simulink model "plantaClosedLoop"  (R2022b)
settings: Solver=VariableStepAuto  StartTime=0.0  StopTime=10.0  MaxStep=0.01  RelTol=1e-3
values from neighbouring files (symbols this model uses):
  d1 = 130.75e-3    (= 0.13075)    [FoundTF.m]    (also in TF.mat)
  d2 = 50.75e-3    (= 0.05075)    [FoundTF.m]    (also in TF.mat)
  DZ = 3    [FoundTF.m]    (also in TF.mat)
  Gden = cell2mat(G.Denominator)    [FoundTF.m]    (also in TF.mat = [1 3.334 0])
  Gnum = cell2mat(G.Numerator)    [FoundTF.m]    (also in TF.mat = [0 0 1.02856666667])
  I = 15e-5    (= 0.00015)    [FoundTF.m]    (also in TF.mat)
  MAX_PWM = 80    [FoundTF.m]    (also in TF.mat)
  thetap = 90    [TF.mat]
  wb = 0.105948    [FoundTF.m]    (also in TF.mat)
  wcp = 0.014145    [FoundTF.m]    (also in TF.mat)
  wm = 0.030411    [FoundTF.m]    (also in TF.mat)
undefined symbols (not defined in the file or in its folder): b, PWM_INPUT
libraries: slpidlib x6
settings Model: Creator=felip  LastModifiedBy=felip

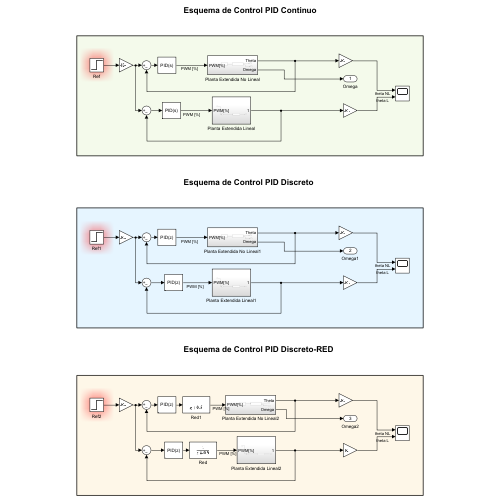
[thumbnail: Simulink's stored preview of the top-level diagram]
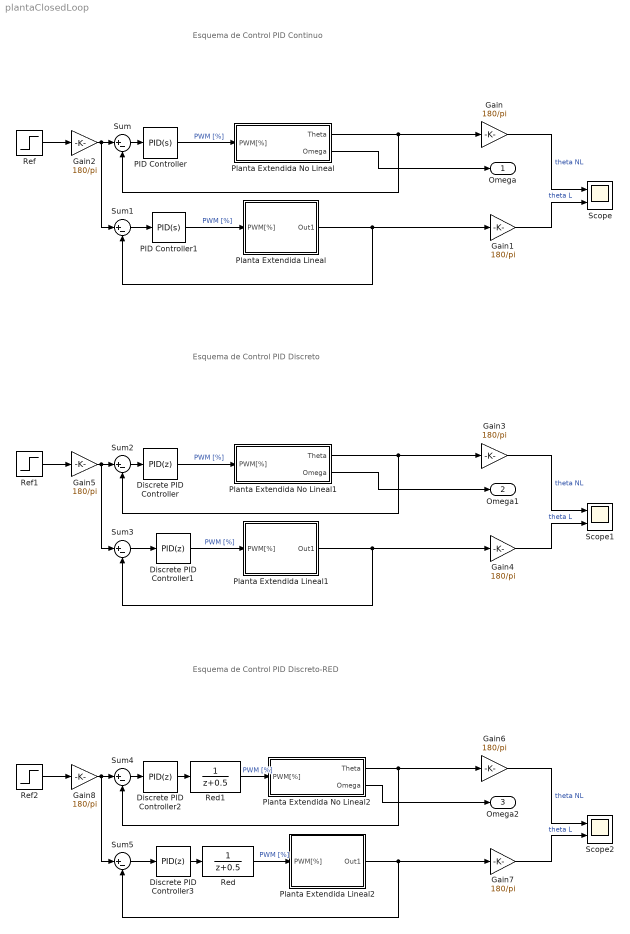
== system plantaClosedLoop ==
  note: Esquema de Control PID Continuo
  note: Esquema de Control PID Discreto
  note: Esquema de Control PID Discreto-RED
  Discrete PID Controller{,1..3} (4 alike) : slpidlib/PID Controller  Controller=PID  Form=Parallel  TimeDomain=Discrete-time  UseExternalTs=off  SampleTime=-1  IntegratorMethod=Forward Euler  FilterMethod=Forward Euler  ControllerParametersSource=internal  P=1  I=1  UseKiTs=off  D=0  N=100  UseFilter=on  TunerSelectOption=Transfer Function Based (PID Tuner App)  InitialConditionSource=internal  InitialConditionForIntegrator=0  InitialConditionForFilter=0  DifferentiatorICPrevScaledInput=0  ExternalReset=none  TrackingMode=off  Kt=1  LimitOutput=off  SatLimitsSource=internal  UpperSaturationLimit=inf  LowerSaturationLimit=-inf  LinearizeAsGain=off  AntiWindupMode=none  Kb=1  LimitIntegrator=off  UpperIntegratorSaturationLimit=inf  LowerIntegratorSaturationLimit=-inf  POutMin=[]  POutMax=[]  IOutMin=[]  IOutMax=[]  DOutMin=[]  DOutMax=[]  NOutMin=[]  NOutMax=[]  SumOutMin=[]  SumOutMax=[]  SaturationOutMin=[]  SaturationOutMax=[]  PParamMin=[]  PParamMax=[]  IParamMin=[]  IParamMax=[]  DParamMin=[]  DParamMax=[]  NParamMin=[]  NParamMax=[]  KbParamMin=[]  KbParamMax=[]  KtParamMin=[]  KtParamMax=[]  KbOutMin=[]  KbOutMax=[]  KtOutMin=[]  KtOutMax=[]  IntegratorOutMin=[]  IntegratorOutMax=[]  FilterOutMin=[]  FilterOutMax=[]  SumI1OutMin=[]  SumI1OutMax=[]  SumI2OutMin=[]  SumI2OutMax=[]  SumI3OutMin=[]  SumI3OutMax=[]  SumI4OutMin=[]  SumI4OutMax=[]  SumDOutMin=[]  SumDOutMax=[]  DifferentiatorOutMin=[]  DifferentiatorOutMax=[]  FilterDiffOutCoefMin=[]  FilterDiffOutCoefMax=[]  ReciprocalOutMin=[]  ReciprocalOutMax=[]  SumDenOutMin=[]  SumDenOutMax=[]  SumNumOutMin=[]  SumNumOutMax=[]  DivideOutMin=[]  DivideOutMax=[]  UdiffTsProdOutMin=[]  UdiffTsProdOutMax=[]  NTsProdOutMin=[]  NTsProdOutMax=[]  UintegralTsProdOutMin=[]  UintegralTsProdOutMax=[]  UngainTsProdOutMin=[]  UngainTsProdOutMax=[]  ClampingZeroOutDataTypeStr=Inherit: Inherit via back propagation  ClampingZeroOutMin=[]  ClampingZeroOutMax=[]  FilterDenConstantOutDataTypeStr=Inherit: Inherit via back propagation  FilterDenConstantOutMin=[]  FilterDenConstantOutMax=[]  PCopyOutDataTypeStr=Inherit: Inherit via back propagation  PCopyOutMin=[]  PCopyOutMax=[]  NCopyOutDataTypeStr=Inherit: Inherit via back propagation  NCopyOutMin=[]  NCopyOutMax=[]  IntegratorContinuousStateAttributes=''  IntegratorStateMustResolveToSignalObject=off  IntegratorRTWStateStorageClass=Auto  FilterContinuousStateAttributes=''  FilterStateMustResolveToSignalObject=off  FilterRTWStateStorageClass=Auto  ParallelPVariant=InternalParameters  IdealPVariant=Disabled  IVariant=InternalParameters  DVariant=InternalParameters  IntegratorVariant=Discrete  SatVariant=Disabled  AWVariant=Passthrough  PCopyVariant=Disabled  TRVariant=Disabled  FdbkBlocksVariant=Forward  IdealPFdbkVariant=Disabled  SatFdbkVariant=Disabled  DerivativeFilterVariant=ForwardEulerFilter  NVariant=InternalParameters  NCopyVariant=Disabled  FilterICVariant=InternalICsFilter  IntegratorICVariant=InternalICs  ExternalResetVariant=Disabled  TRSumVariant=Passthrough  SumFdbkVariant=Disabled  SumVariant=Sum_PID  TsampFilterVariant=InternalTs  TsampNgainVariant=Passthrough  TsampIntegralVariant=Passthrough  ExternalSaturationOutDataTypeStr=Inherit: Same as second input
      settings: LibrarySourceBlock=simulink/Discrete/Discrete PID Controller
  Gain{,1..8} (9 alike) : Gain  Gain=180/pi
  PID Controller : slpidlib/PID Controller  Controller=PID  Form=Parallel  TimeDomain=Continuous-time  UseExternalTs=off  SampleTime=-1  IntegratorMethod=Forward Euler  FilterMethod=Forward Euler  ControllerParametersSource=internal  P=1  I=1  UseKiTs=off  D=0  N=100  UseFilter=on  TunerSelectOption=Transfer Function Based (PID Tuner App)  InitialConditionSource=internal  InitialConditionForIntegrator=0  InitialConditionForFilter=0  DifferentiatorICPrevScaledInput=0  ExternalReset=none  TrackingMode=off  Kt=1  LimitOutput=off  SatLimitsSource=internal  UpperSaturationLimit=inf  LowerSaturationLimit=-inf  LinearizeAsGain=on  AntiWindupMode=none  Kb=1  LimitIntegrator=off  UpperIntegratorSaturationLimit=inf  LowerIntegratorSaturationLimit=-inf  POutMin=[]  POutMax=[]  IOutMin=[]  IOutMax=[]  DOutMin=[]  DOutMax=[]  NOutMin=[]  NOutMax=[]  SumOutMin=[]  SumOutMax=[]  SaturationOutMin=[]  SaturationOutMax=[]  PParamMin=[]  PParamMax=[]  IParamMin=[]  IParamMax=[]  DParamMin=[]  DParamMax=[]  NParamMin=[]  NParamMax=[]  KbParamMin=[]  KbParamMax=[]  KtParamMin=[]  KtParamMax=[]  KbOutMin=[]  KbOutMax=[]  KtOutMin=[]  KtOutMax=[]  IntegratorOutMin=[]  IntegratorOutMax=[]  FilterOutMin=[]  FilterOutMax=[]  SumI1OutMin=[]  SumI1OutMax=[]  SumI2OutMin=[]  SumI2OutMax=[]  SumI3OutMin=[]  SumI3OutMax=[]  SumI4OutMin=[]  SumI4OutMax=[]  SumDOutMin=[]  SumDOutMax=[]  DifferentiatorOutMin=[]  DifferentiatorOutMax=[]  FilterDiffOutCoefMin=[]  FilterDiffOutCoefMax=[]  ReciprocalOutMin=[]  ReciprocalOutMax=[]  SumDenOutMin=[]  SumDenOutMax=[]  SumNumOutMin=[]  SumNumOutMax=[]  DivideOutMin=[]  DivideOutMax=[]  UdiffTsProdOutMin=[]  UdiffTsProdOutMax=[]  NTsProdOutMin=[]  NTsProdOutMax=[]  UintegralTsProdOutMin=[]  UintegralTsProdOutMax=[]  UngainTsProdOutMin=[]  UngainTsProdOutMax=[]  ClampingZeroOutDataTypeStr=Inherit: Inherit via back propagation  ClampingZeroOutMin=[]  ClampingZeroOutMax=[]  FilterDenConstantOutDataTypeStr=Inherit: Inherit via back propagation  FilterDenConstantOutMin=[]  FilterDenConstantOutMax=[]  PCopyOutDataTypeStr=Inherit: Inherit via back propagation  PCopyOutMin=[]  PCopyOutMax=[]  NCopyOutDataTypeStr=Inherit: Inherit via back propagation  NCopyOutMin=[]  NCopyOutMax=[]  IntegratorContinuousStateAttributes=''  IntegratorStateMustResolveToSignalObject=off  IntegratorRTWStateStorageClass=Auto  FilterContinuousStateAttributes=''  FilterStateMustResolveToSignalObject=off  FilterRTWStateStorageClass=Auto  ParallelPVariant=InternalParameters  IdealPVariant=Disabled  IVariant=InternalParameters  DVariant=InternalParameters  IntegratorVariant=Continuous  SatVariant=Disabled  AWVariant=Passthrough  PCopyVariant=Disabled  TRVariant=Disabled  FdbkBlocksVariant=Forward  IdealPFdbkVariant=Disabled  SatFdbkVariant=Disabled  DerivativeFilterVariant=ContFilter  NVariant=InternalParameters  NCopyVariant=Disabled  FilterICVariant=InternalICsFilter  IntegratorICVariant=InternalICs  ExternalResetVariant=Disabled  TRSumVariant=Passthrough  SumFdbkVariant=Disabled  SumVariant=Sum_PID  TsampFilterVariant=InternalTs  TsampNgainVariant=Passthrough  TsampIntegralVariant=Passthrough  ExternalSaturationOutDataTypeStr=Inherit: Same as second input
  PID Controller1 : slpidlib/PID Controller  Controller=PID  Form=Parallel  TimeDomain=Continuous-time  UseExternalTs=off  SampleTime=-1  IntegratorMethod=Forward Euler  FilterMethod=Forward Euler  ControllerParametersSource=internal  P=1  I=1  UseKiTs=off  D=0  N=100  UseFilter=on  TunerSelectOption=Transfer Function Based (PID Tuner App)  InitialConditionSource=internal  InitialConditionForIntegrator=0  InitialConditionForFilter=0  DifferentiatorICPrevScaledInput=0  ExternalReset=none  TrackingMode=off  Kt=1  LimitOutput=off  SatLimitsSource=internal  UpperSaturationLimit=inf  LowerSaturationLimit=-inf  LinearizeAsGain=on  AntiWindupMode=none  Kb=1  LimitIntegrator=off  UpperIntegratorSaturationLimit=inf  LowerIntegratorSaturationLimit=-inf  POutMin=[]  POutMax=[]  IOutMin=[]  IOutMax=[]  DOutMin=[]  DOutMax=[]  NOutMin=[]  NOutMax=[]  SumOutMin=[]  SumOutMax=[]  SaturationOutMin=[]  SaturationOutMax=[]  PParamMin=[]  PParamMax=[]  IParamMin=[]  IParamMax=[]  DParamMin=[]  DParamMax=[]  NParamMin=[]  NParamMax=[]  KbParamMin=[]  KbParamMax=[]  KtParamMin=[]  KtParamMax=[]  KbOutMin=[]  KbOutMax=[]  KtOutMin=[]  KtOutMax=[]  IntegratorOutMin=[]  IntegratorOutMax=[]  FilterOutMin=[]  FilterOutMax=[]  SumI1OutMin=[]  SumI1OutMax=[]  SumI2OutMin=[]  SumI2OutMax=[]  SumI3OutMin=[]  SumI3OutMax=[]  SumI4OutMin=[]  SumI4OutMax=[]  SumDOutMin=[]  SumDOutMax=[]  DifferentiatorOutMin=[]  DifferentiatorOutMax=[]  FilterDiffOutCoefMin=[]  FilterDiffOutCoefMax=[]  ReciprocalOutMin=[]  ReciprocalOutMax=[]  SumDenOutMin=[]  SumDenOutMax=[]  SumNumOutMin=[]  SumNumOutMax=[]  DivideOutMin=[]  DivideOutMax=[]  UdiffTsProdOutMin=[]  UdiffTsProdOutMax=[]  NTsProdOutMin=[]  NTsProdOutMax=[]  UintegralTsProdOutMin=[]  UintegralTsProdOutMax=[]  UngainTsProdOutMin=[]  UngainTsProdOutMax=[]  ClampingZeroOutDataTypeStr=Inherit: Inherit via back propagation  ClampingZeroOutMin=[]  ClampingZeroOutMax=[]  FilterDenConstantOutDataTypeStr=Inherit: Inherit via back propagation  FilterDenConstantOutMin=[]  FilterDenConstantOutMax=[]  PCopyOutDataTypeStr=Inherit: Inherit via back propagation  PCopyOutMin=[]  PCopyOutMax=[]  NCopyOutDataTypeStr=Inherit: Inherit via back propagation  NCopyOutMin=[]  NCopyOutMax=[]  IntegratorContinuousStateAttributes=''  IntegratorStateMustResolveToSignalObject=off  IntegratorRTWStateStorageClass=Auto  FilterContinuousStateAttributes=''  FilterStateMustResolveToSignalObject=off  FilterRTWStateStorageClass=Auto  ParallelPVariant=InternalParameters  IdealPVariant=Disabled  IVariant=InternalParameters  DVariant=InternalParameters  IntegratorVariant=Continuous  SatVariant=Disabled  AWVariant=Passthrough  PCopyVariant=Disabled  TRVariant=Disabled  FdbkBlocksVariant=Forward  IdealPFdbkVariant=Disabled  SatFdbkVariant=Disabled  DerivativeFilterVariant=ContFilter  NVariant=InternalParameters  NCopyVariant=Disabled  FilterICVariant=InternalICsFilter  IntegratorICVariant=InternalICs  ExternalResetVariant=Disabled  TRSumVariant=Passthrough  SumFdbkVariant=Disabled  SumVariant=Sum_PID  TsampFilterVariant=InternalTs  TsampNgainVariant=Passthrough  TsampIntegralVariant=Passthrough  ExternalSaturationOutDataTypeStr=Inherit: Same as second input
  Planta Extendida Lineal : Subsystem
  Planta Extendida Lineal1 : Subsystem
  Planta Extendida Lineal2 : Subsystem
  Planta Extendida No Lineal : Subsystem
  Planta Extendida No Lineal1 : Subsystem
  Planta Extendida No Lineal2 : Subsystem
  Red : DiscreteTransferFcn
  Red1 : DiscreteTransferFcn
  Ref : Step  After=PWM_INPUT  SampleTime=0
  Ref1 : Step  After=PWM_INPUT  SampleTime=0
  Ref2 : Step  After=PWM_INPUT  SampleTime=0
  Scope : Scope  NumInputPorts=2
  Scope1 : Scope  NumInputPorts=2
  Scope2 : Scope  NumInputPorts=2
  Sum{,1..5} (6 alike) : Sum  Inputs=|+-
  Omega : Outport
  Omega1 : Outport  Port=2
  Omega2 : Outport  Port=3
  wires:
  Gain/1 -> Scope/1  "theta NL"
  Gain1/1 -> Scope/2  "theta L"
  Planta Extendida No Lineal/1(Theta) -> Sum/2, Gain/1
  Planta Extendida No Lineal/2(Omega) -> Omega/1
  Planta Extendida Lineal/1(Out1) -> Sum1/2, Gain1/1
  PID Controller/1 -> Planta Extendida No Lineal/1(PWM[%])  "PWM [%]"
  Ref/1 -> Gain2/1
  Gain2/1 -> Sum1/1, Sum/1
  Sum/1 -> PID Controller/1
  PID Controller1/1 -> Planta Extendida Lineal/1(PWM[%])  "PWM [%]"
  Sum1/1 -> PID Controller1/1
  Discrete PID Controller1/1 -> Planta Extendida Lineal1/1(PWM[%])  "PWM [%]"
  Gain5/1 -> Sum3/1, Sum2/1
  Sum3/1 -> Discrete PID Controller1/1
  Discrete PID Controller/1 -> Planta Extendida No Lineal1/1(PWM[%])  "PWM [%]"
  Sum2/1 -> Discrete PID Controller/1
  Planta Extendida No Lineal1/1(Theta) -> Sum2/2, Gain3/1
  Planta Extendida No Lineal1/2(Omega) -> Omega1/1
  Planta Extendida Lineal1/1(Out1) -> Sum3/2, Gain4/1
  Gain4/1 -> Scope1/2  "theta L"
  Ref1/1 -> Gain5/1
  Gain3/1 -> Scope1/1  "theta NL"
  Sum5/1 -> Discrete PID Controller3/1
  Red1/1 -> Planta Extendida No Lineal2/1(PWM[%])  "PWM [%]"
  Red/1 -> Planta Extendida Lineal2/1(PWM[%])  "PWM [%]"
  Gain6/1 -> Scope2/1  "theta NL"
  Ref2/1 -> Gain8/1
  Gain7/1 -> Scope2/2  "theta L"
  Gain8/1 -> Sum5/1, Sum4/1
  Planta Extendida No Lineal2/2(Omega) -> Omega2/1
  Planta Extendida Lineal2/1(Out1) -> Sum5/2, Gain7/1
  Sum4/1 -> Discrete PID Controller2/1
  Planta Extendida No Lineal2/1(Theta) -> Sum4/2, Gain6/1
  Discrete PID Controller2/1 -> Red1/1
  Discrete PID Controller3/1 -> Red/1

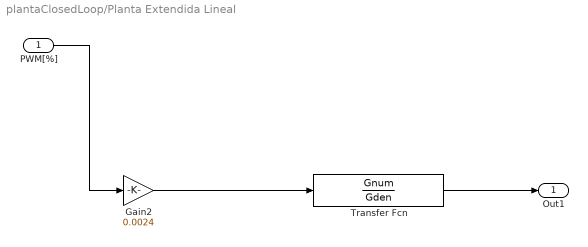
== system plantaClosedLoop/Planta Extendida Lineal ==
  PWM[%] : Inport
  Gain2 : Gain  Gain=0.0024
  Transfer Fcn : TransferFcn  Numerator=Gnum  Denominator=Gden
  Out1 : Outport
  wires:
  Gain2/1 -> Transfer Fcn/1
  PWM[%]/1 -> Gain2/1
  Transfer Fcn/1 -> Out1/1

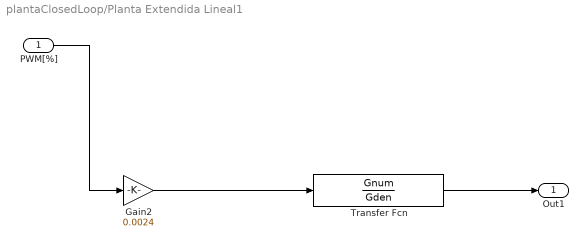
== system plantaClosedLoop/Planta Extendida Lineal1 ==
  PWM[%] : Inport
  Gain2 : Gain  Gain=0.0024
  Transfer Fcn : TransferFcn  Numerator=Gnum  Denominator=Gden
  Out1 : Outport
  wires:
  Gain2/1 -> Transfer Fcn/1
  PWM[%]/1 -> Gain2/1
  Transfer Fcn/1 -> Out1/1

== system plantaClosedLoop/Planta Extendida Lineal2 ==
  PWM[%] : Inport
  Gain2 : Gain  Gain=0.0024
  Transfer Fcn : TransferFcn  Numerator=Gnum  Denominator=Gden
  Out1 : Outport
  wires:
  Gain2/1 -> Transfer Fcn/1
  PWM[%]/1 -> Gain2/1
  Transfer Fcn/1 -> Out1/1

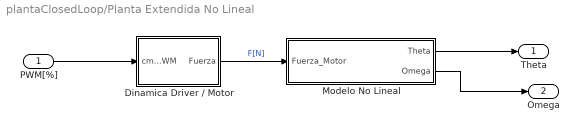
== system plantaClosedLoop/Planta Extendida No Lineal ==
  PWM[%] : Inport
  Dinamica Driver / Motor : Subsystem
  Modelo No Lineal : Subsystem
  Theta : Outport
  Omega : Outport  Port=2
  wires:
  PWM[%]/1 -> Dinamica Driver / Motor/1(cmd_PWM)
  Dinamica Driver / Motor/1(Fuerza) -> Modelo No Lineal/1(Fuerza_Motor)  "F[N]"
  Modelo No Lineal/1(Theta) -> Theta/1
  Modelo No Lineal/2(Omega) -> Omega/1

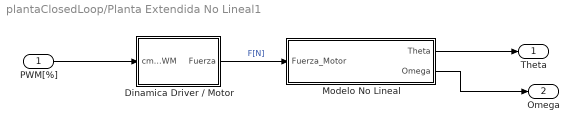
== system plantaClosedLoop/Planta Extendida No Lineal1 ==
  PWM[%] : Inport
  Dinamica Driver / Motor : Subsystem
  Modelo No Lineal : Subsystem
  Theta : Outport
  Omega : Outport  Port=2
  wires:
  PWM[%]/1 -> Dinamica Driver / Motor/1(cmd_PWM)
  Dinamica Driver / Motor/1(Fuerza) -> Modelo No Lineal/1(Fuerza_Motor)  "F[N]"
  Modelo No Lineal/1(Theta) -> Theta/1
  Modelo No Lineal/2(Omega) -> Omega/1

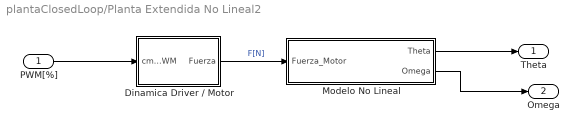
== system plantaClosedLoop/Planta Extendida No Lineal2 ==
  PWM[%] : Inport
  Dinamica Driver / Motor : Subsystem
  Modelo No Lineal : Subsystem
  Theta : Outport
  Omega : Outport  Port=2
  wires:
  PWM[%]/1 -> Dinamica Driver / Motor/1(cmd_PWM)
  Dinamica Driver / Motor/1(Fuerza) -> Modelo No Lineal/1(Fuerza_Motor)  "F[N]"
  Modelo No Lineal/1(Theta) -> Theta/1
  Modelo No Lineal/2(Omega) -> Omega/1

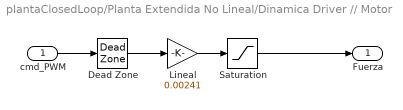
== system plantaClosedLoop/Planta Extendida No Lineal/Dinamica Driver // Motor ==
  cmd_PWM : Inport
  Dead Zone : DeadZone  LowerValue=-DZ  UpperValue=DZ
  Lineal : Gain  Gain=0.00241
  Saturation : Saturate  UpperLimit=MAX_PWM
  Fuerza : Outport
  wires:
  cmd_PWM/1 -> Dead Zone/1
  Saturation/1 -> Fuerza/1
  Dead Zone/1 -> Lineal/1
  Lineal/1 -> Saturation/1

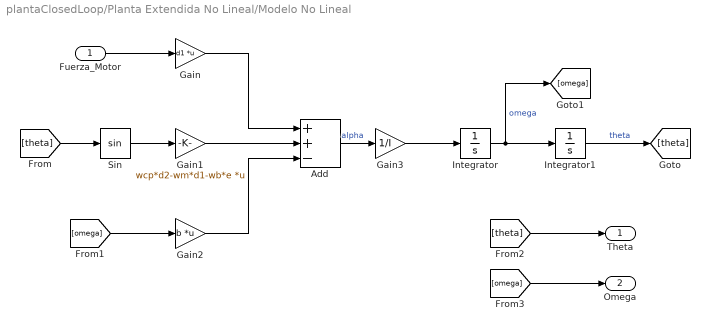
== system plantaClosedLoop/Planta Extendida No Lineal/Modelo No Lineal ==
  Fuerza_Motor : Inport
  Add : Sum  Inputs=++-
  Gain : Gain  Gain=d1  Multiplication=Matrix(K*u)
  Gain1 : Gain  Gain=wcp*d2-wm*d1-wb*e  Multiplication=Matrix(K*u)
  Gain2 : Gain  Gain=b  Multiplication=Matrix(K*u)
  Gain3 : Gain  Gain=1/I
  Integrator : Integrator
  Integrator1 : Integrator  InitialCondition=thetap*pi/180
  Sin : Trigonometry
  Theta : Outport
  Omega : Outport  Port=2
  wires:
  [omega] -> Omega/1
  Gain1/1 -> Add/2
  Integrator/1 -> [omega], Integrator1/1  "omega"
  Fuerza_Motor/1 -> Gain/1
  Integrator1/1 -> [theta]  "theta"
  Gain2/1 -> Add/3
  Gain/1 -> Add/1
  Add/1 -> Gain3/1  "alpha"
  [theta] -> Sin/1
  [omega] -> Gain2/1
  [theta] -> Theta/1
  Sin/1 -> Gain1/1
  Gain3/1 -> Integrator/1

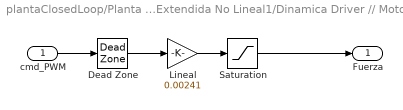
== system plantaClosedLoop/Planta Extendida No Lineal1/Dinamica Driver // Motor ==
  cmd_PWM : Inport
  Dead Zone : DeadZone  LowerValue=-DZ  UpperValue=DZ
  Lineal : Gain  Gain=0.00241
  Saturation : Saturate  UpperLimit=MAX_PWM
  Fuerza : Outport
  wires:
  cmd_PWM/1 -> Dead Zone/1
  Saturation/1 -> Fuerza/1
  Dead Zone/1 -> Lineal/1
  Lineal/1 -> Saturation/1

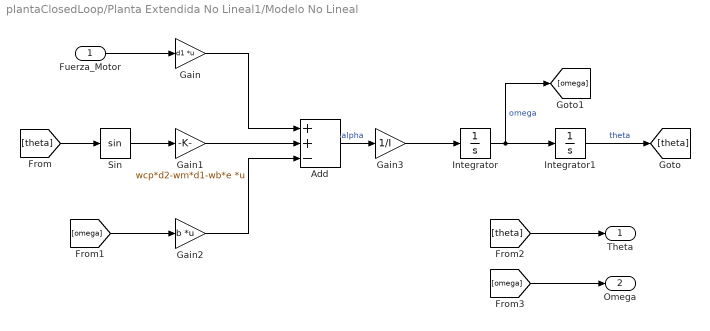
== system plantaClosedLoop/Planta Extendida No Lineal1/Modelo No Lineal ==
  Fuerza_Motor : Inport
  Add : Sum  Inputs=++-
  Gain : Gain  Gain=d1  Multiplication=Matrix(K*u)
  Gain1 : Gain  Gain=wcp*d2-wm*d1-wb*e  Multiplication=Matrix(K*u)
  Gain2 : Gain  Gain=b  Multiplication=Matrix(K*u)
  Gain3 : Gain  Gain=1/I
  Integrator : Integrator
  Integrator1 : Integrator  InitialCondition=thetap*pi/180
  Sin : Trigonometry
  Theta : Outport
  Omega : Outport  Port=2
  wires:
  [omega] -> Omega/1
  Gain1/1 -> Add/2
  Integrator/1 -> [omega], Integrator1/1  "omega"
  Fuerza_Motor/1 -> Gain/1
  Integrator1/1 -> [theta]  "theta"
  Gain2/1 -> Add/3
  Gain/1 -> Add/1
  Add/1 -> Gain3/1  "alpha"
  [theta] -> Sin/1
  [omega] -> Gain2/1
  [theta] -> Theta/1
  Sin/1 -> Gain1/1
  Gain3/1 -> Integrator/1

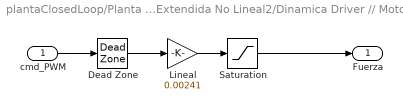
== system plantaClosedLoop/Planta Extendida No Lineal2/Dinamica Driver // Motor ==
  cmd_PWM : Inport
  Dead Zone : DeadZone  LowerValue=-DZ  UpperValue=DZ
  Lineal : Gain  Gain=0.00241
  Saturation : Saturate  UpperLimit=MAX_PWM
  Fuerza : Outport
  wires:
  cmd_PWM/1 -> Dead Zone/1
  Saturation/1 -> Fuerza/1
  Dead Zone/1 -> Lineal/1
  Lineal/1 -> Saturation/1

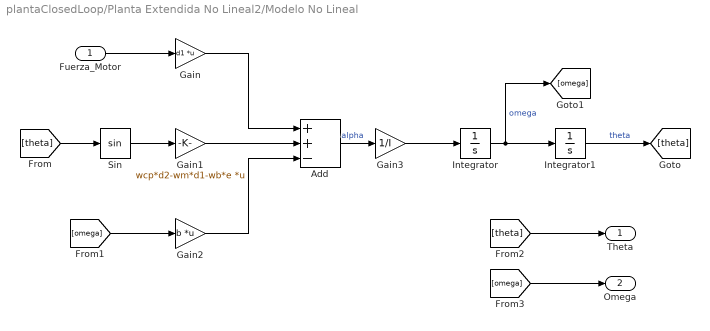
== system plantaClosedLoop/Planta Extendida No Lineal2/Modelo No Lineal ==
  Fuerza_Motor : Inport
  Add : Sum  Inputs=++-
  Gain : Gain  Gain=d1  Multiplication=Matrix(K*u)
  Gain1 : Gain  Gain=wcp*d2-wm*d1-wb*e  Multiplication=Matrix(K*u)
  Gain2 : Gain  Gain=b  Multiplication=Matrix(K*u)
  Gain3 : Gain  Gain=1/I
  Integrator : Integrator
  Integrator1 : Integrator  InitialCondition=thetap*pi/180
  Sin : Trigonometry
  Theta : Outport
  Omega : Outport  Port=2
  wires:
  [omega] -> Omega/1
  Gain1/1 -> Add/2
  Integrator/1 -> [omega], Integrator1/1  "omega"
  Fuerza_Motor/1 -> Gain/1
  Integrator1/1 -> [theta]  "theta"
  Gain2/1 -> Add/3
  Gain/1 -> Add/1
  Add/1 -> Gain3/1  "alpha"
  [theta] -> Sin/1
  [omega] -> Gain2/1
  [theta] -> Theta/1
  Sin/1 -> Gain1/1
  Gain3/1 -> Integrator/1
